simulink model "lab3gravityBC"  (R2023b)
settings: Solver=VariableStepAuto  StartTime=0.0  StopTime=60  RelTol=1e-3
values from neighbouring files (symbols this model uses):
  par = [3, 2, 1, 0.6, 5.0, 5.0, 9.81]    [lab3init.m]
  q0 = [0.785398; -0.785398]    [lab3init.m]
libraries: slpidlib x1
settings Model: Creator=rpl  LastModifiedBy=rpl

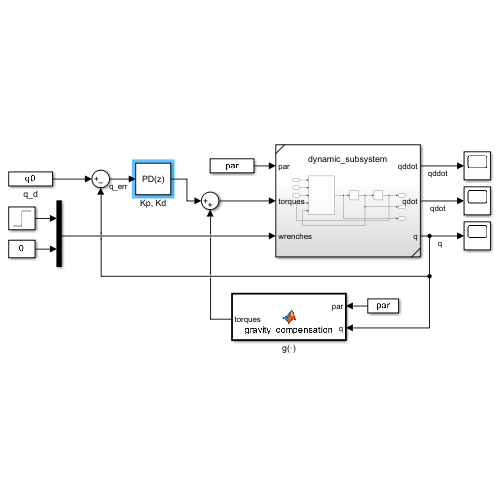
[thumbnail: Simulink's stored preview of the top-level diagram]
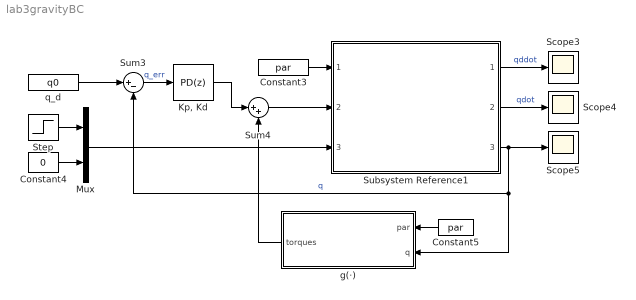
== system lab3gravityBC ==
  Constant3 : Constant  Value=par
  Constant4 : Constant  Value=0
  Constant5 : Constant  Value=par
  "Kp, Kd" : slpidlib/PID Controller  Controller=PD  Form=Parallel  TimeDomain=Discrete-time  UseExternalTs=off  SampleTime=-1  IntegratorMethod=Forward Euler  FilterMethod=Forward Euler  ControllerParametersSource=internal  P=1  I=1  UseKiTs=off  D=1  N=100  UseFilter=on  TunerSelectOption=Transfer Function Based (PID Tuner App)  InitialConditionSource=internal  InitialConditionForIntegrator=0  InitialConditionForFilter=0  DifferentiatorICPrevScaledInput=0  ExternalReset=none  TrackingMode=off  Kt=1  LimitOutput=off  SatLimitsSource=internal  UpperSaturationLimit=inf  LowerSaturationLimit=-inf  LinearizeAsGain=off  AntiWindupMode=none  Kb=1  LimitIntegrator=off  UpperIntegratorSaturationLimit=inf  LowerIntegratorSaturationLimit=-inf  POutMin=[]  POutMax=[]  IOutMin=[]  IOutMax=[]  DOutMin=[]  DOutMax=[]  NOutMin=[]  NOutMax=[]  SumOutMin=[]  SumOutMax=[]  SaturationOutMin=[]  SaturationOutMax=[]  PParamMin=[]  PParamMax=[]  IParamMin=[]  IParamMax=[]  DParamMin=[]  DParamMax=[]  NParamMin=[]  NParamMax=[]  KbParamMin=[]  KbParamMax=[]  KtParamMin=[]  KtParamMax=[]  KbOutMin=[]  KbOutMax=[]  KtOutMin=[]  KtOutMax=[]  IntegratorOutMin=[]  IntegratorOutMax=[]  FilterOutMin=[]  FilterOutMax=[]  SumI1OutMin=[]  SumI1OutMax=[]  SumI2OutMin=[]  SumI2OutMax=[]  SumI3OutMin=[]  SumI3OutMax=[]  SumI4OutMin=[]  SumI4OutMax=[]  SumDOutMin=[]  SumDOutMax=[]  DifferentiatorOutMin=[]  DifferentiatorOutMax=[]  FilterDiffOutCoefMin=[]  FilterDiffOutCoefMax=[]  ReciprocalOutMin=[]  ReciprocalOutMax=[]  SumDenOutMin=[]  SumDenOutMax=[]  SumNumOutMin=[]  SumNumOutMax=[]  DivideOutMin=[]  DivideOutMax=[]  UdiffTsProdOutMin=[]  UdiffTsProdOutMax=[]  NTsProdOutMin=[]  NTsProdOutMax=[]  UintegralTsProdOutMin=[]  UintegralTsProdOutMax=[]  UngainTsProdOutMin=[]  UngainTsProdOutMax=[]  ClampingZeroOutDataTypeStr=Inherit: Inherit via back propagation  ClampingZeroOutMin=[]  ClampingZeroOutMax=[]  FilterDenConstantOutDataTypeStr=Inherit: Inherit via back propagation  FilterDenConstantOutMin=[]  FilterDenConstantOutMax=[]  PCopyOutDataTypeStr=Inherit: Inherit via back propagation  PCopyOutMin=[]  PCopyOutMax=[]  NCopyOutDataTypeStr=Inherit: Inherit via back propagation  NCopyOutMin=[]  NCopyOutMax=[]  IntegratorContinuousStateAttributes=''  IntegratorStateMustResolveToSignalObject=off  IntegratorRTWStateStorageClass=Auto  FilterContinuousStateAttributes=''  FilterStateMustResolveToSignalObject=off  FilterRTWStateStorageClass=Auto  ParallelPVariant=InternalParameters  IdealPVariant=Disabled  IVariant=Disabled  DVariant=InternalParameters  IntegratorVariant=Disabled  SatVariant=Disabled  AWVariant=Disabled  PCopyVariant=Disabled  TRVariant=Disabled  FdbkBlocksVariant=Forward  IdealPFdbkVariant=Disabled  SatFdbkVariant=Disabled  DerivativeFilterVariant=ForwardEulerFilter  NVariant=InternalParameters  NCopyVariant=Disabled  FilterICVariant=InternalICsFilter  IntegratorICVariant=Disabled  ExternalResetVariant=Disabled  TRSumVariant=Passthrough  SumFdbkVariant=Disabled  SumVariant=Sum_PD  TsampFilterVariant=InternalTs  TsampNgainVariant=Passthrough  TsampIntegralVariant=Disabled_SignalSpec  ExternalSaturationOutDataTypeStr=Inherit: Same as second input
      settings: LibrarySourceBlock=simulink/Discrete/Discrete PID Controller
  Mux : Mux  Inputs=2
  Scope3 : Scope
  Scope4 : Scope
  Scope5 : Scope
  Step : Step  Time=2  SampleTime=0
  Subsystem Reference1 : Subsystem  ReferencedSubsystem=dynamic_subsystem
  Sum3 : Sum  Inputs=|+-
  Sum4 : Sum  Inputs=|++
  g(·) : MATLAB Function  TreatAsAtomicUnit=on
  q_d : Constant  Value=q0
  wires:
  Mux/1 -> Subsystem Reference1/3
  Sum4/1 -> Subsystem Reference1/2
  Subsystem Reference1/1 -> Scope3/1  "qddot"
  Subsystem Reference1/2 -> Scope4/1  "qdot"
  Subsystem Reference1/3 -> g(·)/2(q), Sum3/2, Scope5/1  "q"
  Constant3/1 -> Subsystem Reference1/1
  Constant5/1 -> g(·)/1(par)
  q_d/1 -> Sum3/1
  g(·)/1(torques) -> Sum4/2
  Sum3/1 -> "Kp, Kd"/1  "q_err"
  "Kp, Kd"/1 -> Sum4/1
  Constant4/1 -> Mux/2
  Step/1 -> Mux/1

== matlab function lab3gravityBC/g(·) ==
  data: par input; q input; torques output
function torques = gravity_compensation(par, q)

    m1 = par(1);
    m2 = par(2);
    l1 = par(3);
    l2 = par(4);
    g = par(7);

    % sines and cosines
    cq1 = cos(q(1));
    cq12 = cos(q(1)+q(2));
    
    % Calculate g(q)
    g = [(m1+m2)*l1*g*cq1+m2*g*l2*cq12;
          m2*g*l2*cq12];

    torques = g;
